simulink model "Team23_project2_week2"  (R2023b)
settings: Solver=VariableStepAuto  StartTime=0.0  StopTime=201  RelTol=1e-3
values from neighbouring files (symbols this model uses):
  track_radius = 200    [init.m]
undefined symbols (not defined in the file or in its folder): carData
settings Model: Creator=vince  LastModifiedBy=vince

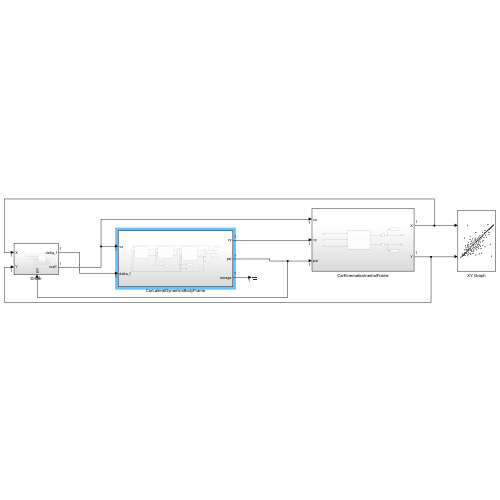
[thumbnail: Simulink's stored preview of the top-level diagram]
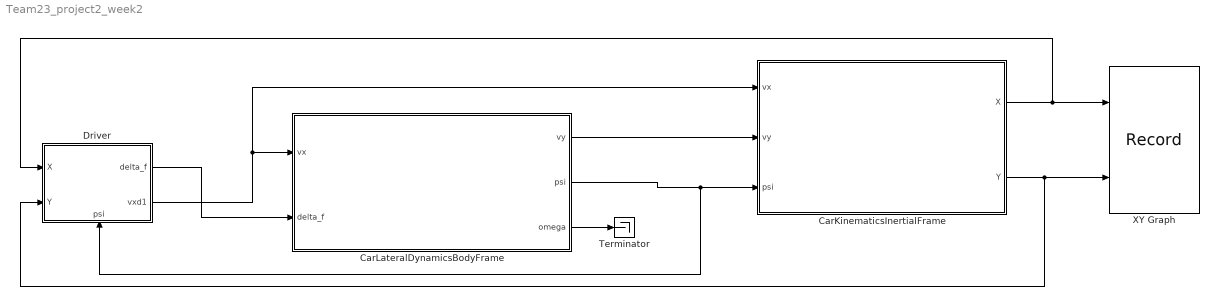
== system Team23_project2_week2 ==
  CarKinematicsInertialFrame : Subsystem
  CarLateralDynamicsBodyFrame : Subsystem
  Driver : Subsystem
      settings: PortSchema="{\"entries\":[{\"content\":{\"sides\":[{\"content\":{\"connectorIds\":[\"In1\",\"In2\"]},\"type\":\"ConnectorPlacement.EquallySpacedRectSide\",\"uuid\":\"94d914a3-e563-41b1-8c36-64a79a2bb31c\"},{\"content\":{\"connectorIds\":[\"Out1\",\"Out2\"],\"side\":\"RIGHT\"},\"type\":\"ConnectorPlacement.EquallySpacedRectSide\",\"uuid\":\"dfe1fa3e-6c4d-45b2-885e-01f359f7acd0\"},{\"content\":{\"side\":\"TOP\"},\"type\":\"ConnectorPlacement.EquallySpacedRectSide\",\"uuid\":\"8261a598-867a-4131-b259-36d0fa5a4b4d\"},{\"content\":{\"connectorIds\":[\"In3\"],\"side\":\"BOTTOM\"},\"type\":\"ConnectorPlacement.EquallySpacedRectSide\",\"uuid\":\"74028213-b440-450a-9cb6-b510a3e405e8\"}]},\"type\":\"ConnectorPlacement.EquallySpacedConnector\",\"uuid\":\"dd8159dc-6811-4628-b85d-54a9a0d0742d\"}],\"packageUris\":[\"http://schema.mathworks.com/mf0/Connector/R2020b\"],\"version\":\"1.0\"}"
  Terminator : Terminator
  XY Graph : Record  FileSettingsInternal="{\"entries\":[{\"content\":{\"excelSettings\":{\"content\":{},\"type\":\"Streamout.ExcelSettings\"}},\"type\":\"Streamout.FileSettingStorage\",\"uuid\":\"\"}],\"packageUris\":[\"http:\\/\\/schema.mathworks.com\\/mf0\\/streamout_blocks\\/R2020a\"],\"version\":\"1.0\"}"  Layout=[1 1]  SignalsInternal="{\"entries\":[{\"content\":{\"signals\":[{\"content\":{\"blockPath\":[],\"dimensions\":[1],\"domain\":\"\",\"lineColor\":\"#a2142f\",\"plots\":[1],\"port\":1,\"signalID\":135,\"signalName\":\"XY Graph:1\"},\"type\":\"RecordBlkView.Signal\",\"uuid\":\"\"},{\"content\":{\"blockPath\":[],\"dimensions\":[1],\"domain\":\"\",\"lineColor\":\"#139fff\",\"plots\":[1],\"port\":2,\"signalID\":138,\"signalName\":\"XY Graph:2\"},\"type\":\"RecordBlkView.Signal\",\"uuid\":\"\"}]},\"type\":\"RecordBlkView.InputSignals\",\"uuid\":\"\"}],\"packageUris\":[\"http:\\/\\/schema.mathworks.com\\/mf0\\/streamout_blocks\\/R2020a\"],\"version\":\"1.0\"}"  VisualizationBindings="{\"xyplotplugin\":{\"info\":[{\"series\":[{\"bindingParametersList\":[{\"parameter\":\"X-Axis\",\"signalID\":135,\"signalName\":\"XY Graph:1\"},{\"parameter\":\"Y-Axis\",\"signalID\":138,\"signalName\":\"XY Graph:2\"}],\"seriesID\":36756}],\"subplotID\":1}]}}"  CompatibilityTag=XY
  wires:
  CarKinematicsInertialFrame/1(X) -> Driver/1(X), XY Graph/1
  CarKinematicsInertialFrame/2(Y) -> Driver/2(Y), XY Graph/2
  CarLateralDynamicsBodyFrame/2(psi) -> CarKinematicsInertialFrame/3(psi), Driver/3(psi)
  CarLateralDynamicsBodyFrame/1(vy) -> CarKinematicsInertialFrame/2(vy)
  CarLateralDynamicsBodyFrame/3(omega) -> Terminator/1
  Driver/2(vxd1) -> CarKinematicsInertialFrame/1(vx), CarLateralDynamicsBodyFrame/1(vx)
  Driver/1(delta_f) -> CarLateralDynamicsBodyFrame/2(delta_f)

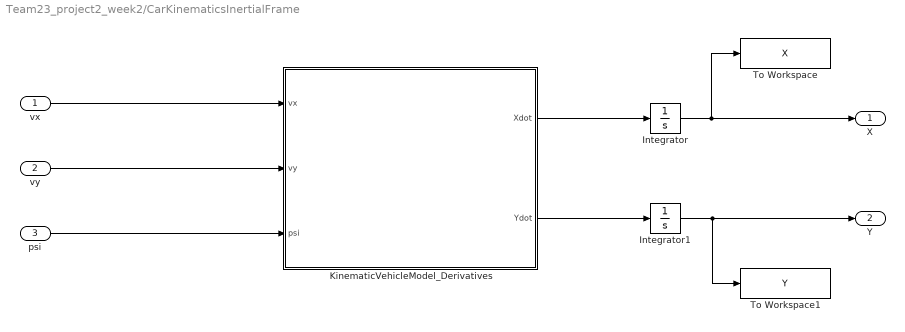
== system Team23_project2_week2/CarKinematicsInertialFrame ==
  vx : Inport
  vy : Inport  Port=2
  psi : Inport  Port=3
  Integrator : Integrator
  Integrator1 : Integrator
  KinematicVehicleModel_Derivatives : MATLAB Function  TreatAsAtomicUnit=on
  To Workspace : ToWorkspace  VariableName=X  SaveFormat=Timeseries  SampleTime=-1
  To Workspace1 : ToWorkspace  VariableName=Y  SaveFormat=Timeseries  SampleTime=-1
  X : Outport
  Y : Outport  Port=2
  wires:
  vx/1 -> KinematicVehicleModel_Derivatives/1(vx)
  vy/1 -> KinematicVehicleModel_Derivatives/2(vy)
  psi/1 -> KinematicVehicleModel_Derivatives/3(psi)
  KinematicVehicleModel_Derivatives/1(Xdot) -> Integrator/1
  KinematicVehicleModel_Derivatives/2(Ydot) -> Integrator1/1
  Integrator/1 -> To Workspace/1, X/1
  Integrator1/1 -> To Workspace1/1, Y/1

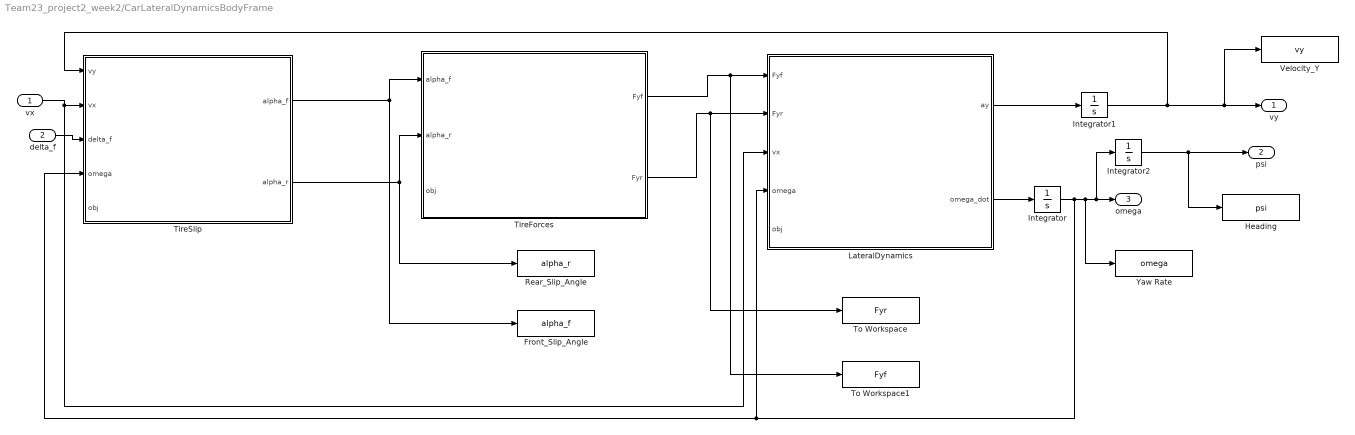
== system Team23_project2_week2/CarLateralDynamicsBodyFrame ==
  vx : Inport
  delta_f : Inport  Port=2
  Front_Slip_Angle : ToWorkspace  VariableName=alpha_f  SaveFormat=Timeseries  SampleTime=-1
  Heading : ToWorkspace  VariableName=psi  SaveFormat=Timeseries  SampleTime=-1
  Integrator : Integrator
  Integrator1 : Integrator
  Integrator2 : Integrator
  LateralDynamics : MATLAB Function  TreatAsAtomicUnit=on
  Rear_Slip_Angle : ToWorkspace  VariableName=alpha_r  SaveFormat=Timeseries  SampleTime=-1
  TireForces : MATLAB Function  TreatAsAtomicUnit=on
  TireSlip : MATLAB Function  TreatAsAtomicUnit=on  mask{obj=carData}
      mask prompts: obj "obj structure"
  To Workspace : ToWorkspace  VariableName=Fyr  SaveFormat=Timeseries  SampleTime=-1
  To Workspace1 : ToWorkspace  VariableName=Fyf  SaveFormat=Timeseries  SampleTime=-1
  Velocity_Y : ToWorkspace  VariableName=vy  SaveFormat=Timeseries  SampleTime=-1
  Yaw Rate : ToWorkspace  VariableName=omega  SaveFormat=Timeseries  SampleTime=-1
  vy : Outport
  psi : Outport  Port=2
  omega : Outport  Port=3
  wires:
  delta_f/1 -> TireSlip/3(delta_f)
  TireSlip/2(alpha_r) -> TireForces/2(alpha_r), Rear_Slip_Angle/1
  TireForces/1(Fyf) -> LateralDynamics/1(Fyf), To Workspace1/1
  TireForces/2(Fyr) -> LateralDynamics/2(Fyr), To Workspace/1
  vx/1 -> LateralDynamics/3(vx), TireSlip/2(vx)
  LateralDynamics/1(ay) -> Integrator1/1
  LateralDynamics/2(omega_dot) -> Integrator/1
  Integrator2/1 -> Heading/1, psi/1
  Integrator1/1 -> TireSlip/1(vy), Velocity_Y/1, vy/1
  Integrator/1 -> LateralDynamics/4(omega), TireSlip/4(omega), Yaw Rate/1, Integrator2/1, omega/1
  TireSlip/1(alpha_f) -> TireForces/1(alpha_f), Front_Slip_Angle/1

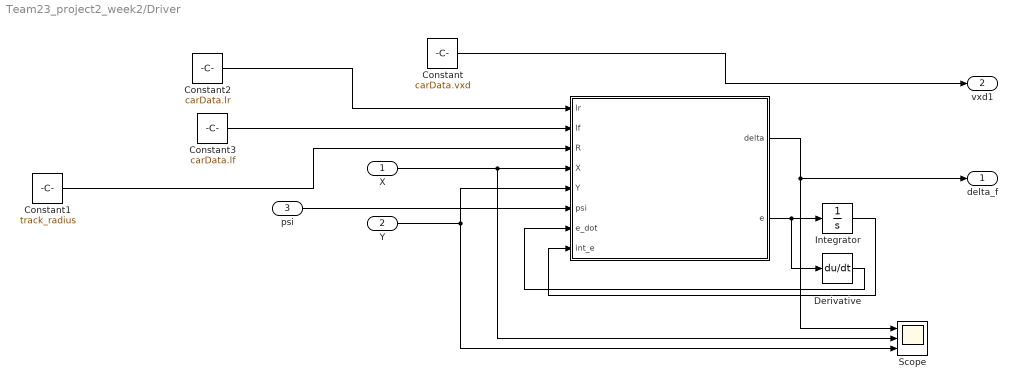
== system Team23_project2_week2/Driver ==
  X : Inport
  Y : Inport  Port=2
  psi : Inport  Port=3
  " " : MATLAB Function  TreatAsAtomicUnit=on
  Constant : Constant  Value=carData.vxd
  Constant1 : Constant  Value=track_radius
  Constant2 : Constant  Value=carData.lr
  Constant3 : Constant  Value=carData.lf
  Derivative : Derivative
  Integrator : Integrator
  Scope : Scope  NumInputPorts=3
  delta_f : Outport
  vxd1 : Outport  Port=2
  wires:
  X/1 -> Scope/2, " "/4(X)
  Y/1 -> Scope/3, " "/5(Y)
  " "/1(delta) -> delta_f/1, Scope/1
  Constant/1 -> vxd1/1
  Constant3/1 -> " "/2(lf)
  Constant2/1 -> " "/1(lr)
  psi/1 -> " "/6(psi)
  " "/2(e) -> Derivative/1, Integrator/1
  Integrator/1 -> " "/8(int_e)
  Derivative/1 -> " "/7(e_dot)
  Constant1/1 -> " "/3(R)

== matlab function Team23_project2_week2/CarKinematicsInertialFrame/KinematicVehicleModel_Derivatives ==
  data: vx input; Xdot output; vy input; psi input; Ydot output
function [Xdot, Ydot] = fcn(vx, vy, psi)
    temp = TF(psi) * [vx;vy];
    Xdot = temp(1);
    Ydot = temp(2);
end

function y = TF(psi)
    y = [cos(psi), -sin(psi); sin(psi), cos(psi)];
end

== matlab function Team23_project2_week2/Driver/  ==
  data: lr input; lf input; R input; X input; delta output; Y input; e output; psi input; e_dot input; int_e input
function [delta, e] = SimplestDriver(lr, lf, R, X, Y, psi, e_dot, int_e)

kp = 0;
kd = 0.05;
ki = 0;

psi_desired=(lr+lf)/R;
e = psi - psi_desired;
PID = kp*e + kd*e_dot + ki*int_e;

delta = PID;

if X >= 900
    if Y < 405
        PID = kp*e + kd*e_dot + ki*int_e;
        delta = PID + psi_desired;
    end
end

if X <= 0
    if Y > 1
        PID = kp*e + kd*e_dot + ki*int_e;
        delta = PID + psi_desired;
    end
end

== matlab function Team23_project2_week2/CarLateralDynamicsBodyFrame/TireSlip ==
  data: vy input; alpha_f output; vx input; delta_f input; omega input; alpha_r output; obj input
function [alpha_f, alpha_r] = fnc(vy, vx, delta_f, omega, obj)

    if abs(vx) > obj.vx_threshold1
        alpha_f = delta_f - (vy + omega * obj.lf) / vx;
        alpha_r = - (vy - omega * obj.lr) / vx;
    else
        alpha_f = 0;
        alpha_r = 0;
    end

end

== matlab function Team23_project2_week2/CarLateralDynamicsBodyFrame/TireForces ==
  data: alpha_f input; Fyf output; alpha_r input; obj input; Fyr output
function [Fyf, Fyr] = fcn(alpha_f, alpha_r, obj)

    Fyf = min(obj.Fyfmax, obj.Calpha_f * alpha_f);
    Fyr = min(obj.Fyrmax, obj.Calpha_r * alpha_r);

end

== matlab function Team23_project2_week2/CarLateralDynamicsBodyFrame/LateralDynamics ==
  data: Fyf input; ay output; Fyr input; vx input; omega input; obj input; omega_dot output
function [ay, omega_dot] = fcn(Fyf, Fyr, vx, omega, obj)

    Fy = Fyf + Fyr;
    ay = Fy / obj.Mass - omega * vx;

    M = Fyf * obj.lf - Fyr * obj.lr;
    omega_dot = M / obj.Inertia;

end
